simulink model "AmpelkreuzungV5_99"  (R2024b)
(part 3 of 3)

    |                 counter7 = counter7 + 1;
    |             otherwise
    |                 disp('error!');
    |         end
    |     end
    | end
  function [autos_auf_spur_fkt, spur_autos] = autos_auf_spur_generieren(spur_autos, timer, autos_auf_spur_fkt):
    | function [autos_auf_spur_fkt, spur_autos] = autos_auf_spur_generieren(spur_autos, timer, autos_auf_spur_fkt)
    |     for i = 1:length(spur_autos)
    |         if (spur_autos(i) < timer && spur_autos(i) ~= 0)
    |             autos_auf_spur_fkt = autos_auf_spur_fkt + 1;
    |             spur_autos(i) = 0;
    |         end
    |     end
    | end
  function [anz_autos_fkt, autos_auf_spur_fkt, counter_neu_fkt, endzeiten] = generiere_gruenphase(spur, laenge, autos_auf_spur_u, counter_alt, start_timer_fkt, endzeiten, startzeiten_fkt, auslastung_fkt, autos_spur1_flag_fkt):
    | function [anz_autos_fkt, autos_auf_spur_fkt, counter_neu_fkt, endzeiten] = generiere_gruenphase(spur, laenge, autos_auf_spur_u, counter_alt, start_timer_fkt, endzeiten, startzeiten_fkt, auslastung_fkt, autos_spur1_flag_fkt) 
    |     if (spur == 2 || spur == 4)  
    |         if laenge < 8.9
    |             anz_autos_fkt = round(0.314739 * power(laenge, 1.2629099));
    |             for i = 1:min([anz_autos_fkt,autos_auf_spur_u])
    |                 endzeiten(counter_alt + i) = start_timer_fkt + nthroot((i / 0.314739), 1.2629099);
    |                 if endzeiten(counter_alt + i) < startzeiten_fkt(counter_alt + i)
    |                     endzeiten(counter_alt + i) = startzeiten_fkt(counter_alt + i);
    |                 end
    |                 if (counter_alt + i) > 1
    |                     if endzeiten(counter_alt + i) < (endzeiten(counter_alt + i - 1) + 0.7)
    |                         endzeiten(counter_alt + i) = endzeiten(counter_alt + i - 1) + 0.7;
    |                     end
    |                 end
    |                 if (endzeiten(counter_alt + i) > start_timer_fkt + laenge)
    |                     endzeiten(counter_alt + i) = 0;
    |                     anz_autos_fkt = anz_autos_fkt - (min(anz_autos_fkt, autos_auf_spur_u) - i + 1);
    |                     break
    |                 end
    |             end
    | 
    |         elseif laenge >= 8.9
    |             anz_autos_fkt = round((laenge - 8.9) / 1.4 + 5);
    |             for i = 1:min([anz_autos_fkt,autos_auf_spur_u])
    |                 if i <= 5
    |                     endzeiten(counter_alt + i) = start_timer_fkt + nthroot((i / 0.314739), 1.2629099);
    |                 else
    |                     endzeiten(counter_alt + i) = start_timer_fkt + 8.9 + (i - 5) * 1.5;
    |                 end             
    |                 if endzeiten(counter_alt + i) < startzeiten_fkt(counter_alt + i)
    |                     endzeiten(counter_alt + i) = startzeiten_fkt(counter_alt + i);
    |                 end
    |                 if (counter_alt + i) > 1
    |                     if endzeiten(counter_alt + i) < (endzeiten(counter_alt + i - 1) + 0.7)
    |                         endzeiten(counter_alt + i) = endzeiten(counter_alt + i - 1) + 0.7;
    |                     end
    |                 end
    |                 if (endzeiten(counter_alt + i) > start_timer_fkt + laenge)
    |                     endzeiten(counter_alt + i) = 0;
    |                     anz_autos_fkt = anz_autos_fkt - (min(anz_autos_fkt, autos_auf_spur_u) - i + 1);
    |                     break
    |                 end                   
    |             end
    |         end
    |          
    |     elseif (spur == 1 || spur == 5 || spur == 6 || spur == 7)
    |         if laenge < 8.3
    |             anz_autos_fkt = round(0.3507674 * power(laenge, 1.2576509));
    |             for i = 1:min([anz_autos_fkt,autos_auf_spur_u])
    |                 endzeiten(counter_alt + i) = start_timer_fkt + nthroot((i / 0.3507674), 1.2576509);
    |                 if endzeiten(counter_alt + i) < startzeiten_fkt(counter_alt + i)
    |                     endzeiten(counter_alt + i) = startzeiten_fkt(counter_alt + i);
    |                 end
    |                 if (counter_alt + i) > 1
    |                     if endzeiten(counter_alt + i) < (endzeiten(counter_alt + i - 1) + 0.9)
    |                         endzeiten(counter_alt + i) = endzeiten(counter_alt + i - 1) + 0.9;
    |                     end
    |                 end
    |                 if (endzeiten(counter_alt + i) > start_timer_fkt + laenge)
    |                     endzeiten(counter_alt + i) = 0;
    |                     anz_autos_fkt = anz_autos_fkt - (min(anz_autos_fkt, autos_auf_spur_u) - i + 1);
    |                     break
    |                 end
    |             end
    | 
    |         elseif laenge >= 8.3
    |             anz_autos_fkt = round((laenge - 8.3) / 1.4 + 5);
    |             for i = 1:min([anz_autos_fkt,autos_auf_spur_u])
    |                 if i<= 5
    |                     endzeiten(counter_alt + i) = start_timer_fkt + nthroot((i / 0.3507674), 1.2576509);
    |                 else
    |                     endzeiten(counter_alt + i) = start_timer_fkt + 8.3 +(i - 5) * 1.4;
    |                 end
    |                 if endzeiten(counter_alt + i) < startzeiten_fkt(counter_alt + i)
    |                     endzeiten(counter_alt + i) = startzeiten_fkt(counter_alt + i);
    |                 end
    |                 if (counter_alt + i) > 1
    |                     if endzeiten(counter_alt + i) < (endzeiten(counter_alt + i - 1) + 0.7)
    |                         endzeiten(counter_alt + i) = endzeiten(counter_alt + i - 1) + 0.7;
    |                     end
    |                 end
    |                 if (endzeiten(counter_alt + i) > start_timer_fkt + laenge)
    |                     endzeiten(counter_alt + i) = 0;
    |                     anz_autos_fkt = anz_autos_fkt - (min(anz_autos_fkt, autos_auf_spur_u) - i + 1);
    |                     break
    |                 end
    |             end
    |         end
    |     
    |     elseif ((auslastung_fkt == 1 || auslastung_fkt == 2) && spur == 3 && autos_spur1_flag_fkt == false)
    |         laenge = laenge - 5;
    |         anz_autos_fkt = round(laenge / 1.5);
    |         for i = 1:min([anz_autos_fkt,autos_auf_spur_u])
    |             if i<= 5
    |                 endzeiten(counter_alt + i) = start_timer_fkt + 5 + nthroot((i / 0.3507674), 1.2576509);
    |             else
    |                 endzeiten(counter_alt + i) = start_timer_fkt + 5 + 8.3 +(i - 5) * 1.4;
    |             end
    |             if endzeiten(counter_alt + i) < startzeiten_fkt(counter_alt + i)
    |                 endzeiten(counter_alt + i) = startzeiten_fkt(counter_alt + i);
    |             end
    |             if (counter_alt + i) > 1
    |                 if endzeiten(counter_alt + i) < (endzeiten(counter_alt + i - 1) + 0.7)
    |                     endzeiten(counter_alt + i) = endzeiten(counter_alt + i - 1) + 0.7;
    |                 end
    |             end
    |             if (endzeiten(counter_alt + i) > start_timer_fkt + 5 + laenge)
    |                 endzeiten(counter_alt + i) = 0;
    |                 anz_autos_fkt = anz_autos_fkt - (min(anz_autos_fkt, autos_auf_spur_u) - i + 1);
    |                 break
    |             end
    |         end
    |     
    |     elseif ( (auslastung_fkt == 1 || auslastung_fkt == 2) && spur == 3 && autos_spur1_flag_fkt == true)
    |         anz_autos_fkt = round(laenge / 1.5);
    |         for i = 1:min([anz_autos_fkt,autos_auf_spur_u])
    |             if i<= 5
    |                 endzeiten(counter_alt + i) = start_timer_fkt + nthroot((i / 0.3507674), 1.2576509);
    |             else
    |                 endzeiten(counter_alt + i) = start_timer_fkt + 8.3 +(i - 5) * 1.4;
    |             end
    |             if endzeiten(counter_alt + i) < startzeiten_fkt(counter_alt + i)
    |                 endzeiten(counter_alt + i) = startzeiten_fkt(counter_alt + i);
    |             end
    |             if (counter_alt + i) > 1
    |                 if endzeiten(counter_alt + i) < (endzeiten(counter_alt + i - 1) + 0.7)
    |                     endzeiten(counter_alt + i) = endzeiten(counter_alt + i - 1) + 0.7;
    |                 end
    |             end
    |             if (endzeiten(counter_alt + i) > start_timer_fkt + laenge)
    |                 endzeiten(counter_alt + i) = 0;
    |                 anz_autos_fkt = anz_autos_fkt - (min(anz_autos_fkt, autos_auf_spur_u) - i + 1);
    |                 break
    |             end
    |         end
    | 
    |     elseif ( auslastung_fkt == 3 && spur == 3 && autos_spur1_flag_fkt == false)
    |         laenge = laenge - 24;
    |         anz_autos_fkt = round(laenge / 1.5);
    |         for i = 1:min([anz_autos_fkt,autos_auf_spur_u])
    |             if i<= 5
    |                 endzeiten(counter_alt + i) = start_timer_fkt + 30 + nthroot((i / 0.3507674), 1.2576509);
    |             else
    |                 endzeiten(counter_alt + i) = start_timer_fkt + 30 + 8.3 +(i - 5) * 1.4;
    |             end
    |             if endzeiten(counter_alt + i) < startzeiten_fkt(counter_alt + i)
    |                 endzeiten(counter_alt + i) = startzeiten_fkt(counter_alt + i);
    |             end
    |             if (counter_alt + i) > 1
    |                 if endzeiten(counter_alt + i) < (endzeiten(counter_alt + i - 1) + 0.7)
    |                     endzeiten(counter_alt + i) = endzeiten(counter_alt + i - 1) + 0.7;
    |                 end
    |             end
    |             if (endzeiten(counter_alt + i) > start_timer_fkt + 30 + laenge)
    |                 endzeiten(counter_alt + i) = 0;
    |                 anz_autos_fkt = anz_autos_fkt - (min(anz_autos_fkt, autos_auf_spur_u) - i + 1);
    |                 break
    |             end
    |         end
    |     
    |     elseif ( auslastung_fkt == 3 && spur == 3 && autos_spur1_flag_fkt == true)
    |         laenge = laenge - 8;
    |         anz_autos_fkt = round(laenge / 1.5);
    |         for i = 1:min([anz_autos_fkt,autos_auf_spur_u])
    |             if i<= 5
    |                 endzeiten(counter_alt + i) = start_timer_fkt + 16 + nthroot((i / 0.3507674), 1.2576509);
    |             else
    |                 endzeiten(counter_alt + i) = start_timer_fkt + 16 + 8.3 +(i - 5) * 1.4;
    |             end
    |             if endzeiten(counter_alt + i) < startzeiten_fkt(counter_alt + i)
    |                 endzeiten(counter_alt + i) = startzeiten_fkt(counter_alt + i);
    |             end
    |             if (counter_alt + i) > 1
    |                 if endzeiten(counter_alt + i) < (endzeiten(counter_alt + i - 1) + 0.7)
    |                     endzeiten(counter_alt + i) = endzeiten(counter_alt + i - 1) + 0.7;
    |                 end
    |             end
    |             if (endzeiten(counter_alt + i) > start_timer_fkt + 16 + laenge)
    |                 endzeiten(counter_alt + i) = 0;
    |                 anz_autos_fkt = anz_autos_fkt - (min(anz_autos_fkt, autos_auf_spur_u) - i + 1);
    |                 break
    |             end
    |         end
    |     
    |     elseif ( auslastung_fkt == 4 && spur == 3 )
    |         laenge = laenge - 35;
    |         anz_autos_fkt = round(laenge / 1.5);
    |         for i = 1:min([anz_autos_fkt,autos_auf_spur_u])
    |             if i<= 5
    |                 endzeiten(counter_alt + i) = start_timer_fkt + 30 + nthroot((i / 0.3507674), 1.2576509);
    |             else
    |                 endzeiten(counter_alt + i) = start_timer_fkt + 30 + 8.3 +(i - 5) * 1.4;
    |             end
    |             if endzeiten(counter_alt + i) < startzeiten_fkt(counter_alt + i)
    |                 endzeiten(counter_alt + i) = startzeiten_fkt(counter_alt + i);
    |             end
    |             if (counter_alt + i) > 1
    |                 if endzeiten(counter_alt + i) < (endzeiten(counter_alt + i - 1) + 0.7)
    |                     endzeiten(counter_alt + i) = endzeiten(counter_alt + i - 1) + 0.7;
    |                 end
    |             end
    |             if (endzeiten(counter_alt + i) > start_timer_fkt + 30 + laenge)
    |                 endzeiten(counter_alt + i) = 0;
    |                 anz_autos_fkt = anz_autos_fkt - (min(anz_autos_fkt, autos_auf_spur_u) - i + 1);
    |                 break
    |             end
    |         end
    | 
    |     elseif ( auslastung_fkt == 5 && spur == 3 )
    |         laenge = laenge - 45;
    |         anz_autos_fkt = round(laenge / 1.5);
    |         for i = 1:min([anz_autos_fkt,autos_auf_spur_u])
    |             if i<= 5
    |                 endzeiten(counter_alt + i) = start_timer_fkt + 30 + nthroot((i / 0.3507674), 1.2576509);
    |             else
    |                 endzeiten(counter_alt + i) = start_timer_fkt + 30 + 8.3 +(i - 5) * 1.4;
    |             end
    |             if endzeiten(counter_alt + i) < startzeiten_fkt(counter_alt + i)
    |                 endzeiten(counter_alt + i) = startzeiten_fkt(counter_alt + i);
    |             end
    |             if (counter_alt + i) > 1
    |                 if endzeiten(counter_alt + i) < (endzeiten(counter_alt + i - 1) + 0.7)
    |                     endzeiten(counter_alt + i) = endzeiten(counter_alt + i - 1) + 0.7;
    |                 end
    |             end
    |             if (endzeiten(counter_alt + i) > start_timer_fkt + 30 + laenge)
    |                 endzeiten(counter_alt + i) = 0;
    |                 anz_autos_fkt = anz_autos_fkt - (min(anz_autos_fkt, autos_auf_spur_u) - i + 1);
    |                 break
    |             end
    |         end
    | 
    |     
    |     else
    |         disp('Fehler')
    |         disp('Fehler')
    |         disp('Fehler')
    |         disp('Fehler')
    |         disp('Fehler')
    |         disp('Fehler')
    |         anz_autos_fkt = 0;
    |     end
    |     
    |     autos_auf_spur_fkt = autos_auf_spur_u - anz_autos_fkt
    |     if autos_auf_spur_fkt < 0
    |         autos_auf_spur_fkt = 0
    |     end
    |     counter_neu_fkt = counter_alt + autos_auf_spur_u - autos_auf_spur_fkt
    |     if counter_neu_fkt < counter_alt
    |         counter_neu_fkt = counter_alt
    |     end
    | end
  function zeit_abstand_fkt = zeit_abstand_aus_auslastung(auslastung_fkt):
    | function zeit_abstand_fkt = zeit_abstand_aus_auslastung(auslastung_fkt)
    |     switch (auslastung_fkt)
    |         case 1
    |             zeit_abstand_fkt = 10
    |         case 2
    |             zeit_abstand_fkt = 4
    |         case 3
    |             zeit_abstand_fkt = 1.6
    |         case 4
    |             zeit_abstand_fkt = 0.95
    |         case 5
    |             zeit_abstand_fkt = 0.84
    |         otherwise
    |             zeit_abstand_fkt = -1000
    |     end
    | end
  function count_spur = countOnwards(time, timeElapsed, spuren):
    | function count_spur = countOnwards(time, timeElapsed, spuren)
    |     count_spur = time;
    |     for i = 1 : length(time)
    |         if spuren(i) == 1
    |             count_spur(i) = count_spur(i) + timeElapsed;
    |         end
    |     end
    | end
  function timer = resetTimer:
    | function timer = resetTimer()
    |     timer = 0;
    | end
  function timer = refresher(startTime, timeElapsed):
    | function timer = refresher(startTime, timeElapsed)
    |     timer = startTime + timeElapsed;
    | end
  function wartezeiten_fkt = berechne_wartezeiten(startzeiten_fkt, endzeiten_fkt, alter_counter_fkt, counter_fkt, wartezeiten_fkt_u):
    | function wartezeiten_fkt = berechne_wartezeiten(startzeiten_fkt, endzeiten_fkt, alter_counter_fkt, counter_fkt, wartezeiten_fkt_u)
    |     wartezeiten_fkt = wartezeiten_fkt_u;
    |     for i = (alter_counter_fkt + 1):counter_fkt
    |         wartezeiten_fkt(i) = endzeiten_fkt(i) - startzeiten_fkt(i);
    |     end
    | end
  function spur_wartezeit_fkt = gesamt_wartezeit_pro_spur(wartezeit_fkt, spur_wartezeit_u, counter_alt_fkt, counter_fkt):
    | function spur_wartezeit_fkt = gesamt_wartezeit_pro_spur(wartezeit_fkt, spur_wartezeit_u, counter_alt_fkt, counter_fkt)
    |     spur_wartezeit_fkt = spur_wartezeit_u;
    |     for i = (1 + counter_alt_fkt:counter_fkt)
    |         spur_wartezeit_fkt = spur_wartezeit_fkt + wartezeit_fkt(i)
    |     end
    | end
    | 
    | %Variablen: wartezeit_fkt: Vektor mit Wartezeiten, spur_wartezeit_u:
    | %Gesamt-Wartezeit auf der Spur bis zu dem Zeitpunkt
  function gesamtwartezeit_fkt = berechne_gesamtwartezeit(ges_wartezeit1_fkt, ges_wartezeit2_fkt, ges_wartezeit3_fkt, ges_wartezeit4_fkt, ges_wartezeit5_fkt, ges_wartezeit6_fkt, ges_wartezeit7_fkt):
    | function gesamtwartezeit_fkt = berechne_gesamtwartezeit(ges_wartezeit1_fkt, ges_wartezeit2_fkt, ges_wartezeit3_fkt, ges_wartezeit4_fkt, ges_wartezeit5_fkt, ges_wartezeit6_fkt, ges_wartezeit7_fkt)
    |     gesamtwartezeit_fkt = ges_wartezeit1_fkt + ges_wartezeit2_fkt + ges_wartezeit3_fkt + ges_wartezeit4_fkt + ges_wartezeit5_fkt + ges_wartezeit6_fkt + ges_wartezeit7_fkt;
    | end
  function gesamte_autos_fkt = berechne_gesamte_autos(counter1_fkt, counter2_fkt, counter3_fkt, counter4_fkt, counter5_fkt, counter6_fkt, counter7_fkt):
    | function gesamte_autos_fkt = berechne_gesamte_autos(counter1_fkt, counter2_fkt, counter3_fkt, counter4_fkt, counter5_fkt, counter6_fkt, counter7_fkt)
    |     gesamte_autos_fkt = counter1_fkt + counter2_fkt + counter3_fkt + counter4_fkt + counter5_fkt + counter6_fkt + counter7_fkt;
    | end
